simulink library "EqM"  (R2024b)
settings: Solver=VariableStepAuto  StartTime=0.0  StopTime=10.0  RelTol=1e-3
undefined symbols (not defined in the file): g
libraries: $bdroot x1
settings Model: Creator=ada09  LastModifiedBy=ada09

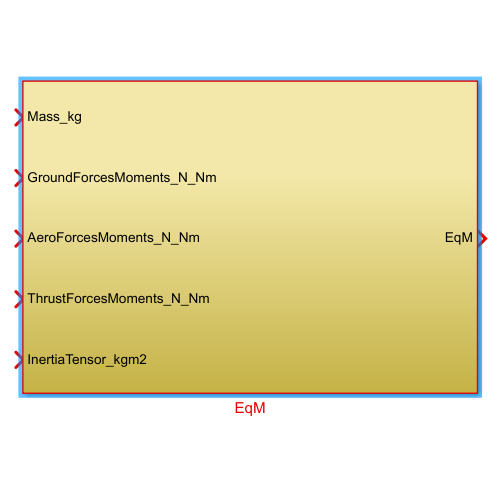
[thumbnail: Simulink's stored preview of the top-level diagram]
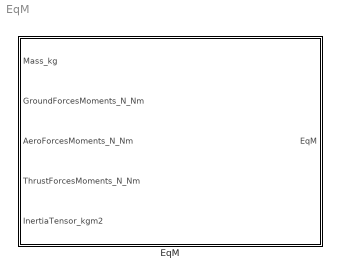
== system EqM ==
  EqM : Subsystem

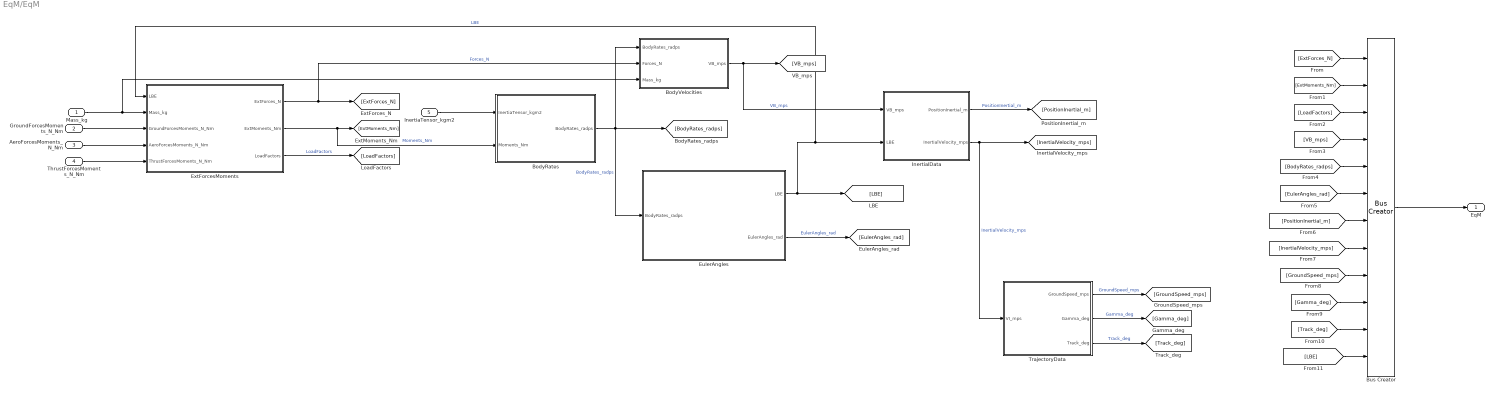
== system EqM/EqM ==
  Mass_kg : Inport
  GroundForcesMoments_N_Nm : Inport  Port=2
  AeroForcesMoments_N_Nm : Inport  Port=3
  ThrustForcesMoments_N_Nm : Inport  Port=4
  InertiaTensor_kgm2 : Inport  Port=5
  BodyRates : Subsystem
  BodyVelocities : Subsystem
  Bus Creator : BusCreator  Inputs=12
  EulerAngles : Subsystem
  ExtForcesMoments : Subsystem
  InertialData : Subsystem
  TrajectoryData : Subsystem
  EqM : Outport
  wires:
  [LBE] -> Bus Creator/12
  [VB_mps] -> Bus Creator/4
  ExtForcesMoments/1(ExtForces_N) -> [ExtForces_N], BodyVelocities/2(Forces_N)  "Forces_N"
  EulerAngles/1(LBE) -> ExtForcesMoments/1(LBE), InertialData/2(LBE), [LBE]  "LBE"
  BodyRates/1(BodyRates_radps) -> BodyVelocities/1(BodyRates_radps), [BodyRates_radps], EulerAngles/1(BodyRates_radps)  "BodyRates_radps"
  [Track_deg] -> Bus Creator/11
  InertiaTensor_kgm2/1 -> BodyRates/1(InertiaTensor_kgm2)
  [GroundSpeed_mps] -> Bus Creator/9
  AeroForcesMoments_N_Nm/1 -> ExtForcesMoments/4(AeroForcesMoments_N_Nm)
  EulerAngles/2(EulerAngles_rad) -> [EulerAngles_rad]  "EulerAngles_rad"
  ExtForcesMoments/2(ExtMoments_Nm) -> [ExtMoments_Nm], BodyRates/2(Moments_Nm)  "Moments_Nm"
  ThrustForcesMoments_N_Nm/1 -> ExtForcesMoments/5(ThrustForcesMoments_N_Nm)
  TrajectoryData/1(GroundSpeed_mps) -> [GroundSpeed_mps]  "GroundSpeed_mps"
  GroundForcesMoments_N_Nm/1 -> ExtForcesMoments/3(GroundForcesMoments_N_Nm)
  BodyVelocities/1(VB_mps) -> [VB_mps], InertialData/1(VB_mps)  "VB_mps"
  [Gamma_deg] -> Bus Creator/10
  [InertialVelocity_mps] -> Bus Creator/8
  [ExtMoments_Nm] -> Bus Creator/2
  Mass_kg/1 -> ExtForcesMoments/2(Mass_kg), BodyVelocities/3(Mass_kg)
  ExtForcesMoments/3(LoadFactors) -> [LoadFactors]  "LoadFactors"
  [LoadFactors] -> Bus Creator/3
  InertialData/2(InertialVelocity_mps) -> [InertialVelocity_mps], TrajectoryData/1(VI_mps)  "InertialVelocity_mps"
  [ExtForces_N] -> Bus Creator/1
  InertialData/1(PositionInertial_m) -> [PositionInertial_m]  "PositionInertial_m"
  [BodyRates_radps] -> Bus Creator/5
  TrajectoryData/3(Track_deg) -> [Track_deg]  "Track_deg"
  [EulerAngles_rad] -> Bus Creator/6
  [PositionInertial_m] -> Bus Creator/7
  TrajectoryData/2(Gamma_deg) -> [Gamma_deg]  "Gamma_deg"
  Bus Creator/1 -> EqM/1

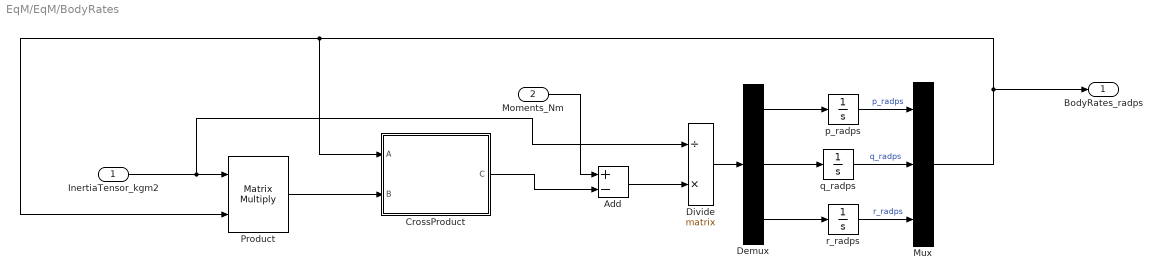
== system EqM/EqM/BodyRates ==
  InertiaTensor_kgm2 : Inport
  Moments_Nm : Inport  Port=2
  Add : Sum  Inputs=+-
  CrossProduct : Subsystem
  Demux : Demux  Outputs=3
  Divide : Product  Inputs=/*  Multiplication=Matrix(*)
  Mux : Mux  Inputs=3
  Product : Product  Multiplication=Matrix(*)
  p_radps : Integrator  ContinuousStateAttributes='p_radps'
  q_radps : Integrator  ContinuousStateAttributes='q_radps'
  r_radps : Integrator  ContinuousStateAttributes='r_radps'
  BodyRates_radps : Outport
  wires:
  Product/1 -> CrossProduct/2(B)
  Demux/2 -> q_radps/1
  Demux/1 -> p_radps/1
  Moments_Nm/1 -> Add/1
  Add/1 -> Divide/2
  Mux/1 -> BodyRates_radps/1, CrossProduct/1(A), Product/2
  InertiaTensor_kgm2/1 -> Divide/1, Product/1
  CrossProduct/1(C) -> Add/2
  r_radps/1 -> Mux/3  "r_radps"
  q_radps/1 -> Mux/2  "q_radps"
  Divide/1 -> Demux/1
  p_radps/1 -> Mux/1  "p_radps"
  Demux/3 -> r_radps/1

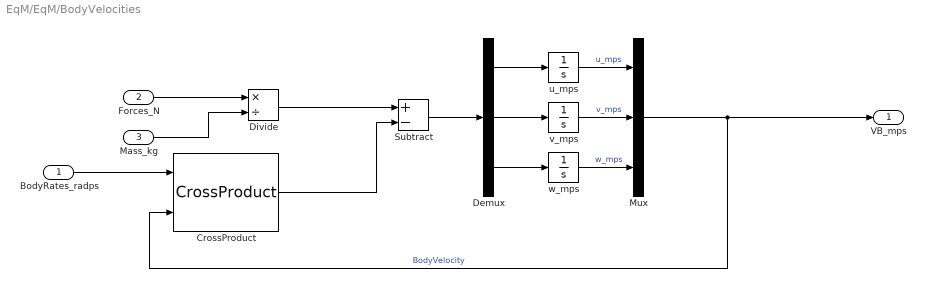
== system EqM/EqM/BodyVelocities ==
  BodyRates_radps : Inport
  Forces_N : Inport  Port=2
  Mass_kg : Inport  Port=3
  CrossProduct : $bdroot/EqM/BodyRates/CrossProduct  SystemSampleTime=-1  VariantActivationTime=update diagram  AllowFlexibleInterface=on  Latency=0  AutoFrameSizeCalculation=off
  Demux : Demux  Outputs=3
  Divide : Product  Inputs=*/
  Mux : Mux  Inputs=3
  Subtract : Sum  Inputs=+-
  u_mps : Integrator  ContinuousStateAttributes='u_mps'
  v_mps : Integrator  ContinuousStateAttributes='v_mps'
  w_mps : Integrator  ContinuousStateAttributes='w_mps'
  VB_mps : Outport
  wires:
  Demux/1 -> u_mps/1
  u_mps/1 -> Mux/1  "u_mps"
  Demux/3 -> w_mps/1
  Demux/2 -> v_mps/1
  BodyRates_radps/1 -> CrossProduct/1
  Subtract/1 -> Demux/1
  Divide/1 -> Subtract/1
  v_mps/1 -> Mux/2  "v_mps"
  Mux/1 -> VB_mps/1, CrossProduct/2  "BodyVelocity"
  Mass_kg/1 -> Divide/2
  w_mps/1 -> Mux/3  "w_mps"
  Forces_N/1 -> Divide/1
  CrossProduct/1 -> Subtract/2

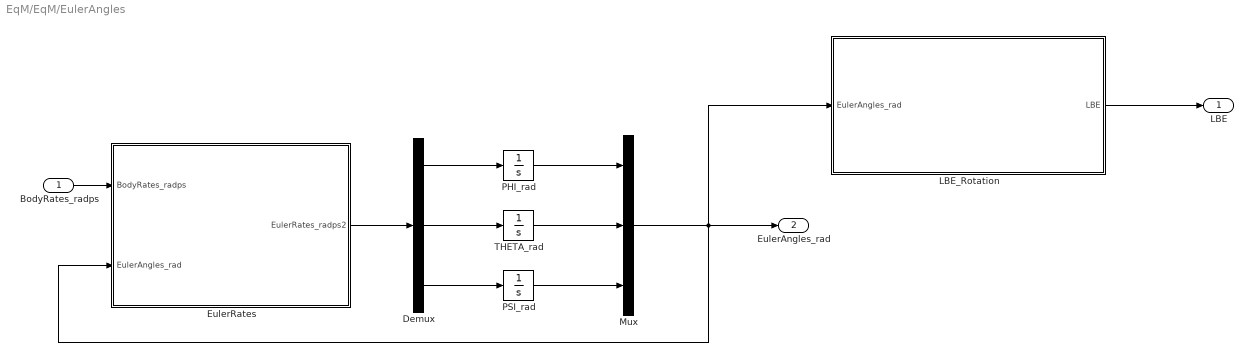
== system EqM/EqM/EulerAngles ==
  BodyRates_radps : Inport
  Demux : Demux  Outputs=3
  EulerRates : Subsystem
  LBE_Rotation : Subsystem
  Mux : Mux  Inputs=3
  PHI_rad : Integrator  ContinuousStateAttributes='PHI_rad'
  PSI_rad : Integrator  ContinuousStateAttributes='PSI_rad'
  THETA_rad : Integrator  ContinuousStateAttributes='THETA_rad'
  LBE : Outport
  EulerAngles_rad : Outport  Port=2
  wires:
  Demux/1 -> PHI_rad/1
  PHI_rad/1 -> Mux/1
  PSI_rad/1 -> Mux/3
  LBE_Rotation/1(LBE) -> LBE/1
  Demux/3 -> PSI_rad/1
  Mux/1 -> EulerRates/2(EulerAngles_rad), EulerAngles_rad/1, LBE_Rotation/1(EulerAngles_rad)
  THETA_rad/1 -> Mux/2
  Demux/2 -> THETA_rad/1
  EulerRates/1(EulerRates_radps2) -> Demux/1
  BodyRates_radps/1 -> EulerRates/1(BodyRates_radps)

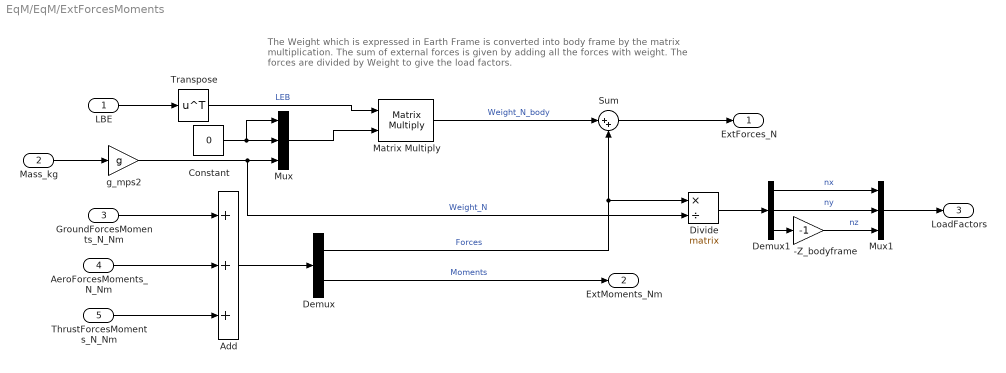
== system EqM/EqM/ExtForcesMoments ==
  note: The Weight which is expressed in Earth Frame is converted into body frame by the matrix multiplication. The sum of external forces is given by adding all the forces with weight. The forces are divided by Weight to give the load factors.
  LBE : Inport
  Mass_kg : Inport  Port=2
  GroundForcesMoments_N_Nm : Inport  Port=3
  AeroForcesMoments_N_Nm : Inport  Port=4
  ThrustForcesMoments_N_Nm : Inport  Port=5
  -Z_bodyframe : Gain  Gain=-1
  Add : Sum  Inputs=+++
  Constant : Constant  Value=0
  Demux : Demux  Outputs=2
  Demux1 : Demux  Outputs=3
  Divide : Product  Inputs=*/  Multiplication=Matrix(*)
  Matrix Multiply : Product  Multiplication=Matrix(*)
  Mux : Mux  Inputs=3
  Mux1 : Mux  Inputs=3
  Sum : Sum  Inputs=|++
  Transpose : Math  Operator=transpose
  g_mps2 : Gain  Gain=g
  ExtForces_N : Outport
  ExtMoments_Nm : Outport  Port=2
  LoadFactors : Outport  Port=3
  wires:
  Mux/1 -> Matrix Multiply/2
  Demux1/3 -> -Z_bodyframe/1
  Demux1/1 -> Mux1/1  "nx"
  Add/1 -> Demux/1
  g_mps2/1 -> Divide/2, Mux/3  "Weight_N"
  Demux/2 -> ExtMoments_Nm/1  "Moments"
  Transpose/1 -> Matrix Multiply/1  "LEB"
  Demux/1 -> Sum/2, Divide/1  "Forces"
  Demux1/2 -> Mux1/2  "ny"
  ThrustForcesMoments_N_Nm/1 -> Add/3
  Constant/1 -> Mux/1, Mux/2
  -Z_bodyframe/1 -> Mux1/3  "nz"
  Divide/1 -> Demux1/1
  Sum/1 -> ExtForces_N/1
  GroundForcesMoments_N_Nm/1 -> Add/1
  AeroForcesMoments_N_Nm/1 -> Add/2
  LBE/1 -> Transpose/1
  Mux1/1 -> LoadFactors/1
  Mass_kg/1 -> g_mps2/1
  Matrix Multiply/1 -> Sum/1  "Weight_N_body"

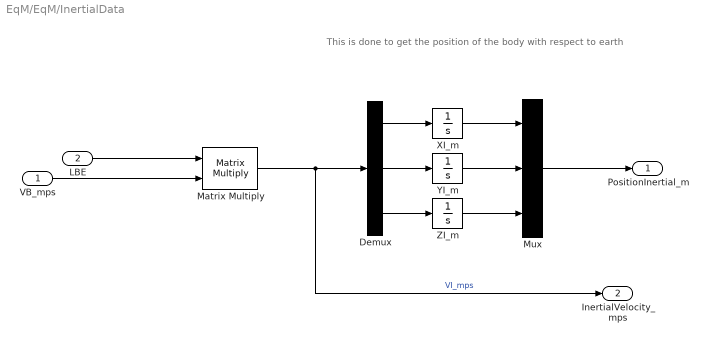
== system EqM/EqM/InertialData ==
  note: This is done to get the position of the body with respect to earth
  VB_mps : Inport
  LBE : Inport  Port=2
  Demux : Demux  Outputs=3
  Matrix Multiply : Product  Multiplication=Matrix(*)
  Mux : Mux  Inputs=3
  XI_m : Integrator  ContinuousStateAttributes='XI_m'
  YI_m : Integrator  ContinuousStateAttributes='YI_m'
  ZI_m : Integrator  ContinuousStateAttributes='ZI_m'
  PositionInertial_m : Outport
  InertialVelocity_mps : Outport  Port=2
  wires:
  XI_m/1 -> Mux/1
  Demux/2 -> YI_m/1
  Matrix Multiply/1 -> InertialVelocity_mps/1, Demux/1  "VI_mps"
  Demux/3 -> ZI_m/1
  ZI_m/1 -> Mux/3
  Demux/1 -> XI_m/1
  Mux/1 -> PositionInertial_m/1
  YI_m/1 -> Mux/2
  VB_mps/1 -> Matrix Multiply/2
  LBE/1 -> Matrix Multiply/1

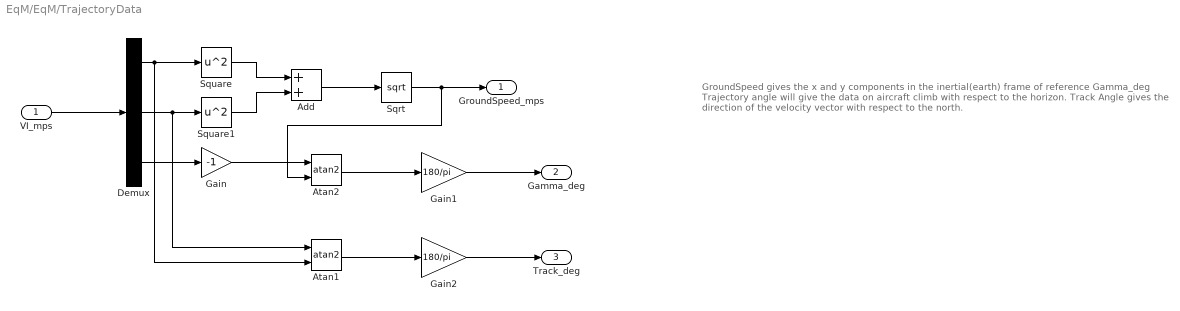
== system EqM/EqM/TrajectoryData ==
  note: GroundSpeed gives the x and y components in the inertial(earth) frame of reference
      | Gamma_deg Trajectory angle will give the data on aircraft climb with respect to the horizon.
      | Track Angle gives the direction of the velocity vector with respect to the north.
  VI_mps : Inport
  Add : Sum
  Atan1 : Trigonometry  Operator=atan2
  Atan2 : Trigonometry  Operator=atan2
  Demux : Demux  Outputs=3
  Gain : Gain  Gain=-1
  Gain1 : Gain  Gain=180/pi
  Gain2 : Gain  Gain=180/pi
  Sqrt : Sqrt
  Square : Math  Operator=square
  Square1 : Math  Operator=square
  GroundSpeed_mps : Outport
  Gamma_deg : Outport  Port=2
  Track_deg : Outport  Port=3
  wires:
  Square/1 -> Add/1
  Demux/2 -> Atan1/1, Square1/1
  Gain1/1 -> Gamma_deg/1
  Demux/1 -> Atan1/2, Square/1
  Add/1 -> Sqrt/1
  Demux/3 -> Gain/1
  Atan2/1 -> Gain1/1
  Gain2/1 -> Track_deg/1
  Square1/1 -> Add/2
  Atan1/1 -> Gain2/1
  Sqrt/1 -> GroundSpeed_mps/1, Atan2/2
  Gain/1 -> Atan2/1
  VI_mps/1 -> Demux/1

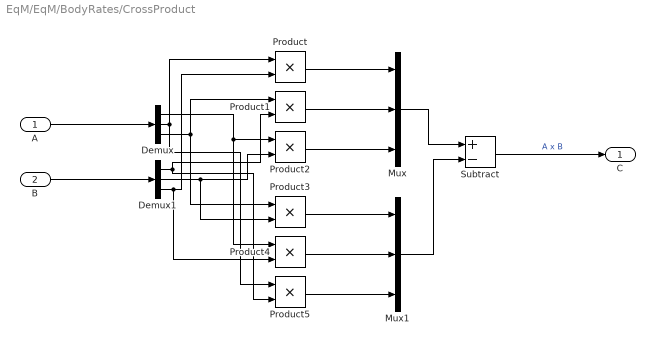
== system EqM/EqM/BodyRates/CrossProduct ==
  A : Inport
  B : Inport  Port=2
  Demux : Demux  Outputs=3
  Demux1 : Demux  Outputs=3
  Mux : Mux  Inputs=3
  Mux1 : Mux  Inputs=3
  Product{,1..5} (6 alike) : Product
  Subtract : Sum  Inputs=+-
  C : Outport
  wires:
  Demux/1 -> Product4/1, Product2/1
  Product3/1 -> Mux1/1
  Demux1/3 -> Product4/2, Product/2
  Demux/2 -> Product5/1, Product/1
  Product5/1 -> Mux1/3
  Demux1/1 -> Product5/2, Product1/2
  Demux/3 -> Product3/1, Product1/1
  Mux/1 -> Subtract/1
  B/1 -> Demux1/1
  Demux1/2 -> Product3/2, Product2/2
  Product4/1 -> Mux1/2
  Product2/1 -> Mux/3
  Product/1 -> Mux/1
  Product1/1 -> Mux/2
  Mux1/1 -> Subtract/2
  A/1 -> Demux/1
  Subtract/1 -> C/1  "A x B"

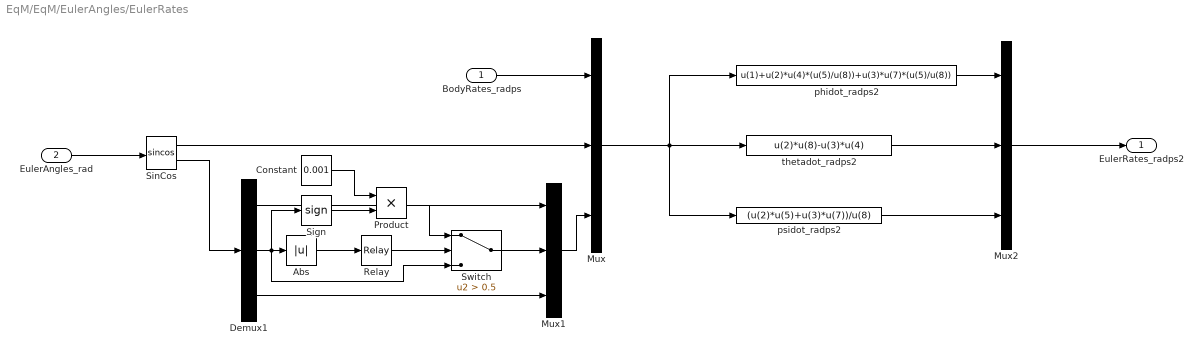
== system EqM/EqM/EulerAngles/EulerRates ==
  BodyRates_radps : Inport
  EulerAngles_rad : Inport  Port=2
  Abs : Abs  SaturateOnIntegerOverflow=off
  Constant : Constant  Value=0.001
  Demux1 : Demux  Outputs=3
  Mux : Mux  Inputs=3
  Mux1 : Mux  Inputs=3
  Mux2 : Mux  Inputs=3
  Product : Product
  Relay : Relay  OnSwitchValue=0.001  OffSwitchValue=0  OnOutputValue=0  OffOutputValue=1
  Sign : Signum
  SinCos : Trigonometry  Operator=sincos
  Switch : Switch  Criteria=u2 > Threshold  Threshold=0.5  SaturateOnIntegerOverflow=off  InputSameDT=off
  phidot_radps2 : Fcn  Expr=u(1)+u(2)*u(4)*(u(5)/u(8))+u(3)*u(7)*(u(5)/u(8))
  psidot_radps2 : Fcn  Expr=(u(2)*u(5)+u(3)*u(7))/u(8)
  thetadot_radps2 : Fcn  Expr=u(2)*u(8)-u(3)*u(4)
  EulerRates_radps2 : Outport
  wires:
  Sign/1 -> Product/2
  Relay/1 -> Switch/2
  Mux/1 -> psidot_radps2/1, phidot_radps2/1, thetadot_radps2/1
  Demux1/3 -> Mux1/3
  EulerAngles_rad/1 -> SinCos/1
  SinCos/2 -> Demux1/1
  thetadot_radps2/1 -> Mux2/2
  BodyRates_radps/1 -> Mux/1
  SinCos/1 -> Mux/2
  Abs/1 -> Relay/1
  Demux1/2 -> Sign/1, Switch/3, Abs/1
  Product/1 -> Switch/1
  Constant/1 -> Product/1
  Mux1/1 -> Mux/3
  Demux1/1 -> Mux1/1
  Switch/1 -> Mux1/2
  phidot_radps2/1 -> Mux2/1
  psidot_radps2/1 -> Mux2/3
  Mux2/1 -> EulerRates_radps2/1

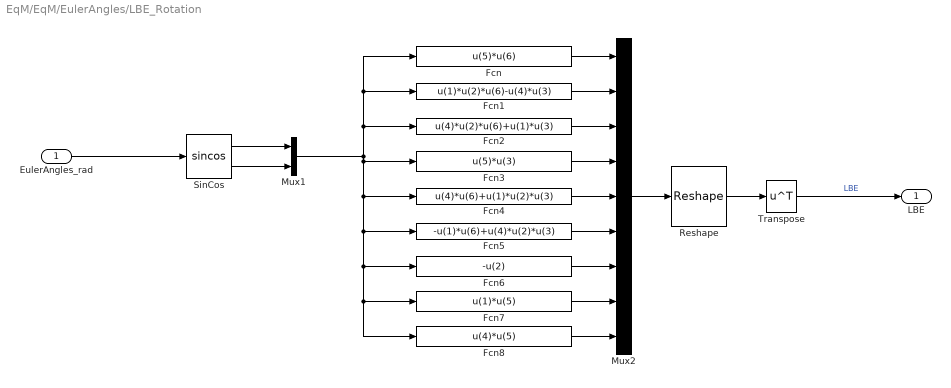
== system EqM/EqM/EulerAngles/LBE_Rotation ==
  EulerAngles_rad : Inport
  Fcn : Fcn  Expr=u(5)*u(6)
  Fcn1 : Fcn  Expr=u(1)*u(2)*u(6)-u(4)*u(3)
  Fcn2 : Fcn  Expr=u(4)*u(2)*u(6)+u(1)*u(3)
  Fcn3 : Fcn  Expr=u(5)*u(3)
  Fcn4 : Fcn  Expr=u(4)*u(6)+u(1)*u(2)*u(3)
  Fcn5 : Fcn  Expr=-u(1)*u(6)+u(4)*u(2)*u(3)
  Fcn6 : Fcn  Expr=-u(2)
  Fcn7 : Fcn  Expr=u(1)*u(5)
  Fcn8 : Fcn  Expr=u(4)*u(5)
  Mux1 : Mux  Inputs=2
  Mux2 : Mux  Inputs=9
  Reshape : Reshape  OutputDimensionality=Customize  OutputDimensions=[3,3]
  SinCos : Trigonometry  Operator=sincos
  Transpose : Math  Operator=transpose
  LBE : Outport
  wires:
  Fcn/1 -> Mux2/1
  Fcn2/1 -> Mux2/3
  Mux1/1 -> Fcn3/1, Fcn8/1, Fcn7/1, Fcn6/1, Fcn5/1, Fcn4/1, Fcn2/1, Fcn1/1, Fcn/1
  Transpose/1 -> LBE/1  "LBE"
  Reshape/1 -> Transpose/1
  Fcn6/1 -> Mux2/7
  SinCos/1 -> Mux1/1
  Fcn1/1 -> Mux2/2
  Fcn4/1 -> Mux2/5
  Fcn7/1 -> Mux2/8
  EulerAngles_rad/1 -> SinCos/1
  Fcn3/1 -> Mux2/4
  Fcn8/1 -> Mux2/9
  SinCos/2 -> Mux1/2
  Mux2/1 -> Reshape/1
  Fcn5/1 -> Mux2/6
